simulink model "L13_exercise"  (R2023b)
settings: Solver=FixedStepDiscrete  StartTime=0.0  StopTime=600  FixedStep=0.1  RelTol=1e-3
values from neighbouring files (symbols this model uses):
  Ki = 2    [visualize.m]
  Kp = 1    [visualize.m]
  LP = c2d(tf([N], [1 N]), 0.1)    [visualize.m]
libraries: simulink x8, slpidlib x1
settings Model: PauseTimes=190  Creator=tbcigcb  LastModifiedBy=vojta
settings OptimizationCC: ReuseModelBlockBuffer=off

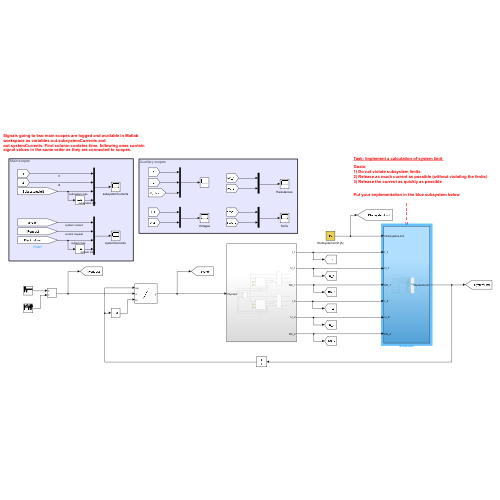
[thumbnail: Simulink's stored preview of the top-level diagram]
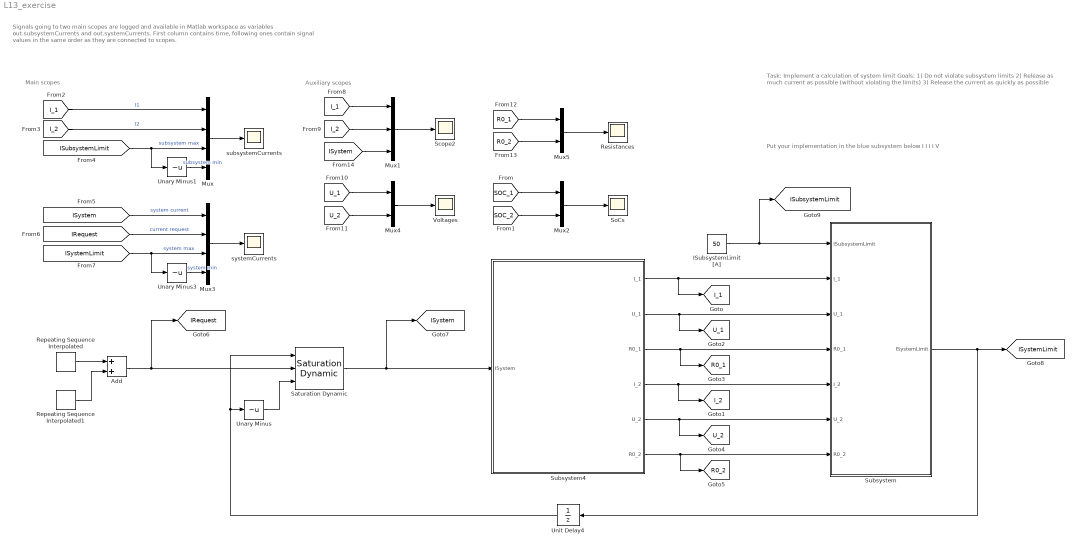
== system L13_exercise ==
  note: Task: Implement a calculation of system limit
      |
      | Goals:
      | 1) Do not violate subsystem limits
      | 2) Release as much current as possible (without violating the limits)
      | 3) Release the current as quickly as possible
  note: Signals going to two main scopes are logged and available in Matlab workspace as variables out.subsystemCurrents and out.systemCurrents. First column contains time, following ones contain signal values in the same order as they are connected to scopes.
  note: Put your implementation in the blue subsystem below
      |
      | I
      | I
      | I
      | I
      | V
  note: Main scopes
  note: Auxiliary scopes
  Add : Sum
  ISubsystemLimit [A] : Constant  Value=50  SampleTime=0.1
  Mux : Mux
  Mux1 : Mux  Inputs=3
  Mux2 : Mux  Inputs=2
  Mux3 : Mux
  Mux4 : Mux  Inputs=2
  Mux5 : Mux  Inputs=2
  Repeating Sequence Interpolated : simulink/Sources/Repeating Sequence Interpolated  OutValues=200*[0 0 1 0 -1 0 0]+0.01  TimeValues=[0 10 20 30 40 50 150]  LookUpMeth=Interpolation-Use End Values  tsamp=0.1  OutMin=[]  OutMax=[]  OutDataTypeStr=double  OutputDataTypeScalingMode=double  OutDataType=fixdt(0,8)  OutScaling=2^-10
  Repeating Sequence Interpolated1 : simulink/Sources/Repeating Sequence Interpolated  OutValues=120*[0 1 0 -1 0 0.5 1 -1 1 0.7 0]+0.01  TimeValues=[0 60 70 80 90 100 110 120 130 140 150]  LookUpMeth=Use Input Below  tsamp=0.1  OutMin=[]  OutMax=[]  OutDataTypeStr=double  OutputDataTypeScalingMode=double  OutDataType=fixdt(0,8)  OutScaling=2^-10
  Resistances : Scope
  Saturation Dynamic : simulink/Discontinuities/Saturation Dynamic  OutMin=[]  OutMax=[]  OutDataTypeStr=Inherit: Same as second input  OutDataType=fixdt(1, 16)  OutScaling=2^-10  DoSatur=off
  Scope2 : Scope
  SoCs : Scope
  Subsystem : Subsystem
  Subsystem4 : Subsystem
  Unary Minus : UnaryMinus
  Unary Minus1 : UnaryMinus
  Unary Minus3 : UnaryMinus
  Unit Delay4 : UnitDelay  InitialCondition=100  SampleTime=-1  HasFrameUpgradeWarning=on
  Voltages : Scope
  subsystemCurrents : Scope
  systemCurrents : Scope
  tag scope: IRequest=global, ISubsystemLimit=global, ISystem=global, ISystemLimit=global, I_1=global, I_2=global, R0_1=global, R0_2=global, U_1=global, U_2=global
  wires:
  Subsystem/1(ISystemLimit) -> [ISystemLimit], Unit Delay4/1
  Unit Delay4/1 -> Saturation Dynamic/1, Unary Minus/1
  Unary Minus/1 -> Saturation Dynamic/3
  Saturation Dynamic/1 -> [ISystem], Subsystem4/1(ISystem)
  Add/1 -> [IRequest], Saturation Dynamic/2
  Mux/1 -> subsystemCurrents/1
  Repeating Sequence Interpolated1/1 -> Add/2
  Repeating Sequence Interpolated/1 -> Add/1
  ISubsystemLimit [A]/1 -> [ISubsystemLimit], Subsystem/1(ISubsystemLimit)
  Unary Minus1/1 -> Mux/4  "subsystem min"
  [SOC_1] -> Mux2/1
  [SOC_2] -> Mux2/2
  Mux2/1 -> SoCs/1
  Subsystem4/1(I_1) -> [I_1], Subsystem/2(I_1)
  Subsystem4/2(U_1) -> [U_1], Subsystem/3(U_1)
  Subsystem4/3(R0_1) -> [R0_1], Subsystem/4(R0_1)
  Subsystem4/4(I_2) -> [I_2], Subsystem/5(I_2)
  Subsystem4/5(U_2) -> [U_2], Subsystem/6(U_2)
  Subsystem4/6(R0_2) -> [R0_2], Subsystem/7(R0_2)
  [I_1] -> Mux/1  "I1"
  [I_2] -> Mux/2  "I2"
  [ISubsystemLimit] -> Unary Minus1/1, Mux/3  "subsystem max"
  Unary Minus3/1 -> Mux3/4  "system min"
  Mux3/1 -> systemCurrents/1
  [IRequest] -> Mux3/2  "current request"
  [ISystemLimit] -> Unary Minus3/1, Mux3/3  "system max"
  [ISystem] -> Mux3/1  "system current"
  Mux1/1 -> Scope2/1
  [I_2] -> Mux1/2
  [I_1] -> Mux1/1
  [U_1] -> Mux4/1
  [U_2] -> Mux4/2
  Mux4/1 -> Voltages/1
  Mux5/1 -> Resistances/1
  [R0_2] -> Mux5/2
  [R0_1] -> Mux5/1
  [ISystem] -> Mux1/3

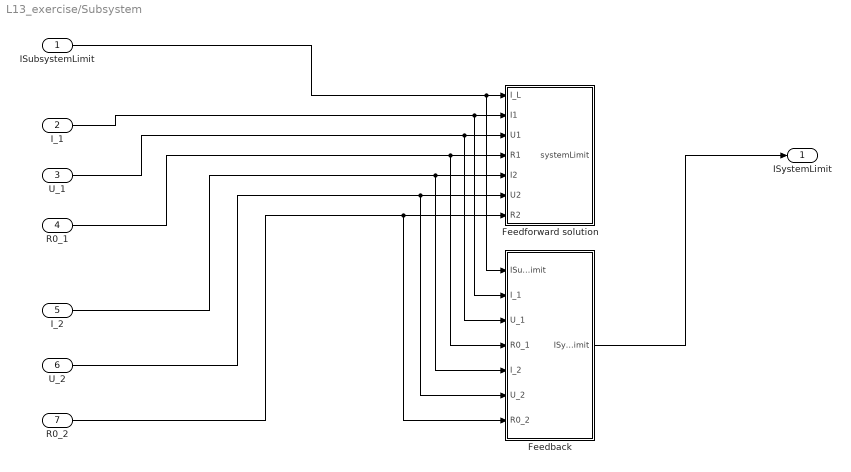
== system L13_exercise/Subsystem ==
  ISubsystemLimit : Inport
  I_1 : Inport  Port=2
  U_1 : Inport  Port=3
  R0_1 : Inport  Port=4
  I_2 : Inport  Port=5
  U_2 : Inport  Port=6
  R0_2 : Inport  Port=7
  Feedback : Subsystem
  Feedforward solution : MATLAB Function  TreatAsAtomicUnit=on
  ISystemLimit : Outport
  wires:
  ISubsystemLimit/1 -> Feedback/1(ISubsystemLimit), Feedforward solution/1(I_L)
  U_1/1 -> Feedback/3(U_1), Feedforward solution/3(U1)
  I_1/1 -> Feedback/2(I_1), Feedforward solution/2(I1)
  R0_1/1 -> Feedback/4(R0_1), Feedforward solution/4(R1)
  I_2/1 -> Feedback/5(I_2), Feedforward solution/5(I2)
  U_2/1 -> Feedback/6(U_2), Feedforward solution/6(U2)
  R0_2/1 -> Feedback/7(R0_2), Feedforward solution/7(R2)
  Feedback/1(ISystemLimit) -> ISystemLimit/1

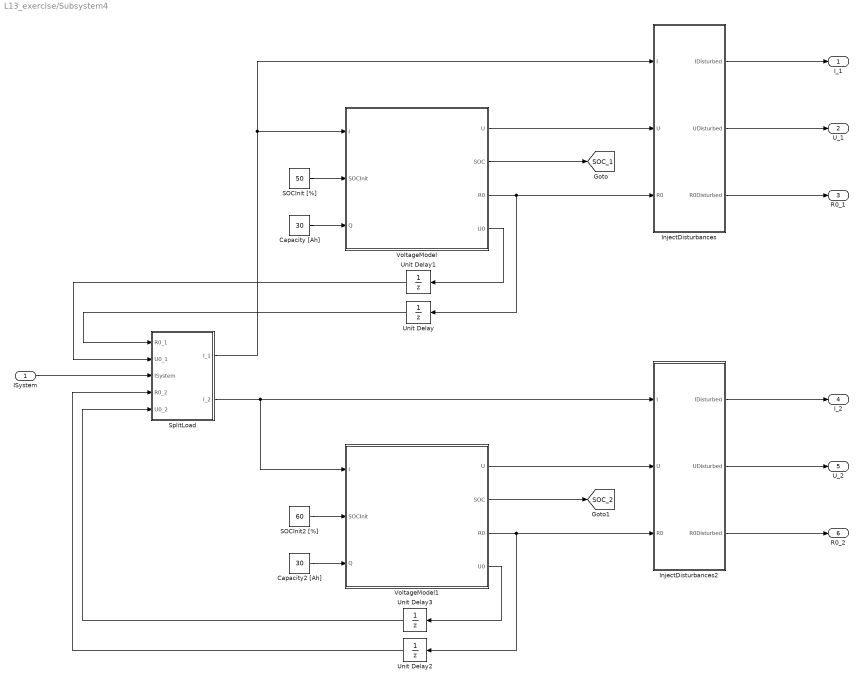
== system L13_exercise/Subsystem4 ==
  ISystem : Inport
  Capacity [Ah] : Constant  Value=30
  Capacity2 [Ah] : Constant  Value=30
  InjectDisturbances : Subsystem
  InjectDisturbances2 : Subsystem
  SOCInit [%] : Constant  Value=50
  SOCInit2 [%] : Constant  Value=60
  SplitLoad : Subsystem
  Unit Delay : UnitDelay  InitialCondition=1  SampleTime=-1  HasFrameUpgradeWarning=on
  Unit Delay1 : UnitDelay  SampleTime=-1  HasFrameUpgradeWarning=on
  Unit Delay2 : UnitDelay  InitialCondition=1  SampleTime=-1  HasFrameUpgradeWarning=on
  Unit Delay3 : UnitDelay  SampleTime=-1  HasFrameUpgradeWarning=on
  VoltageModel : Subsystem
  VoltageModel1 : Subsystem
  I_1 : Outport
  U_1 : Outport  Port=2
  R0_1 : Outport  Port=3
  I_2 : Outport  Port=4
  U_2 : Outport  Port=5
  R0_2 : Outport  Port=6
  tag scope: SOC_1=global, SOC_2=global
  wires:
  SOCInit2 [%]/1 -> VoltageModel1/2(SOCInit)
  SplitLoad/1(I_1) -> InjectDisturbances/1(I), VoltageModel/1(I)
  VoltageModel/4(U0) -> Unit Delay1/1
  Unit Delay1/1 -> SplitLoad/2(U0_1)
  Unit Delay3/1 -> SplitLoad/5(U0_2)
  SplitLoad/2(I_2) -> VoltageModel1/1(I), InjectDisturbances2/1(I)
  Unit Delay/1 -> SplitLoad/1(R0_1)
  VoltageModel1/3(R0) -> InjectDisturbances2/3(R0), Unit Delay2/1
  Unit Delay2/1 -> SplitLoad/4(R0_2)
  SOCInit [%]/1 -> VoltageModel/2(SOCInit)
  VoltageModel/3(R0) -> InjectDisturbances/3(R0), Unit Delay/1
  VoltageModel1/4(U0) -> Unit Delay3/1
  Capacity2 [Ah]/1 -> VoltageModel1/3(Q)
  Capacity [Ah]/1 -> VoltageModel/3(Q)
  ISystem/1 -> SplitLoad/3(ISystem)
  VoltageModel/2(SOC) -> [SOC_1]
  VoltageModel1/2(SOC) -> [SOC_2]
  InjectDisturbances/1(IDisturbed) -> I_1/1
  VoltageModel/1(U) -> InjectDisturbances/2(U)
  InjectDisturbances/2(UDisturbed) -> U_1/1
  InjectDisturbances/3(R0Disturbed) -> R0_1/1
  VoltageModel1/1(U) -> InjectDisturbances2/2(U)
  InjectDisturbances2/3(R0Disturbed) -> R0_2/1
  InjectDisturbances2/2(UDisturbed) -> U_2/1
  InjectDisturbances2/1(IDisturbed) -> I_2/1

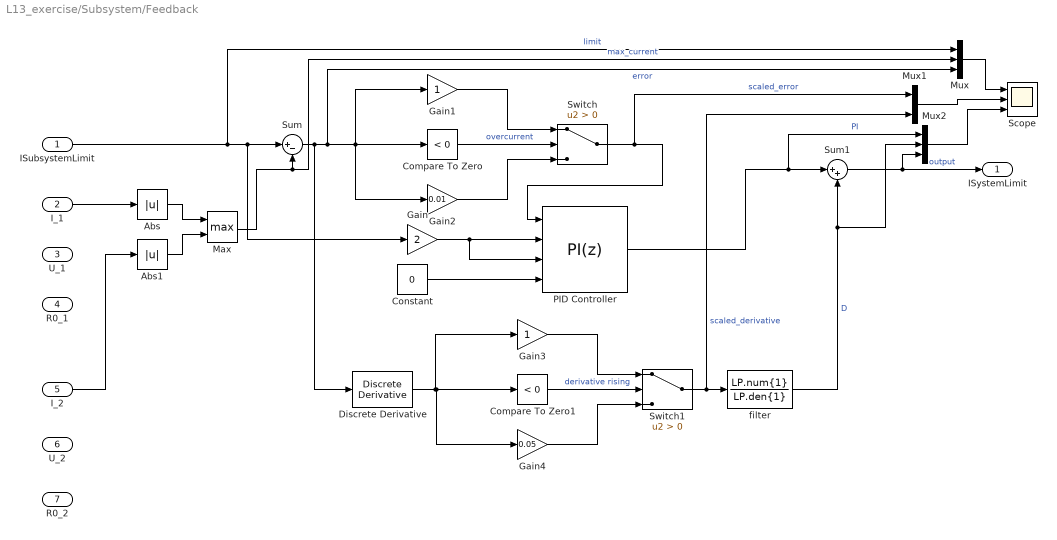
== system L13_exercise/Subsystem/Feedback ==
  ISubsystemLimit : Inport
  I_1 : Inport  Port=2
  U_1 : Inport  Port=3
  R0_1 : Inport  Port=4
  I_2 : Inport  Port=5
  U_2 : Inport  Port=6
  R0_2 : Inport  Port=7
  Abs : Abs  SaturateOnIntegerOverflow=off
  Abs1 : Abs  SaturateOnIntegerOverflow=off
  Compare To Zero : simulink/Logic and Bit Operations/Compare To Zero  relop=<  OutDataTypeStr=boolean
  Compare To Zero1 : simulink/Logic and Bit Operations/Compare To Zero  relop=<  OutDataTypeStr=boolean
  Constant : Constant  Value=0
  Discrete Derivative : simulink/Discrete/Discrete Derivative  gainval=Kd  ICPrevScaledInput=0.0  OutMin=[]  OutMax=[]  OutDataType=fixdt(1, 16)  OutScaling=2^-10  DoSatur=off
  Gain : Gain  Gain=2
  Gain1 : Gain
  Gain2 : Gain  Gain=0.01
  Gain3 : Gain
  Gain4 : Gain  Gain=0.05
  Max : MinMax  Function=max  Inputs=2
  Mux : Mux  Inputs=3
  Mux1 : Mux  Inputs=2
  Mux2 : Mux  Inputs=3
  PID Controller : slpidlib/PID Controller  Controller=PI  Form=Parallel  TimeDomain=Discrete-time  UseExternalTs=off  SampleTime=-1  IntegratorMethod=Forward Euler  FilterMethod=Forward Euler  ControllerParametersSource=internal  P=Kp  I=Ki  UseKiTs=off  D=0  N=100  UseFilter=on  TunerSelectOption=Transfer Function Based (PID Tuner App)  InitialConditionSource=external  InitialConditionForIntegrator=0  InitialConditionForFilter=0  DifferentiatorICPrevScaledInput=0  ExternalReset=none  TrackingMode=off  Kt=1  LimitOutput=on  SatLimitsSource=external  UpperSaturationLimit=inf  LowerSaturationLimit=-inf  LinearizeAsGain=on  AntiWindupMode=clamping  Kb=1  LimitIntegrator=off  UpperIntegratorSaturationLimit=inf  LowerIntegratorSaturationLimit=-inf  POutMin=[]  POutMax=[]  IOutMin=[]  IOutMax=[]  DOutMin=[]  DOutMax=[]  NOutMin=[]  NOutMax=[]  SumOutMin=[]  SumOutMax=[]  SaturationOutMin=[]  SaturationOutMax=[]  PParamMin=[]  PParamMax=[]  IParamMin=[]  IParamMax=[]  DParamMin=[]  DParamMax=[]  NParamMin=[]  NParamMax=[]  KbParamMin=[]  KbParamMax=[]  KtParamMin=[]  KtParamMax=[]  KbOutMin=[]  KbOutMax=[]  KtOutMin=[]  KtOutMax=[]  IntegratorOutMin=[]  IntegratorOutMax=[]  FilterOutMin=[]  FilterOutMax=[]  SumI1OutMin=[]  SumI1OutMax=[]  SumI2OutMin=[]  SumI2OutMax=[]  SumI3OutMin=[]  SumI3OutMax=[]  SumI4OutMin=[]  SumI4OutMax=[]  SumDOutMin=[]  SumDOutMax=[]  DifferentiatorOutMin=[]  DifferentiatorOutMax=[]  FilterDiffOutCoefMin=[]  FilterDiffOutCoefMax=[]  ReciprocalOutMin=[]  ReciprocalOutMax=[]  SumDenOutMin=[]  SumDenOutMax=[]  SumNumOutMin=[]  SumNumOutMax=[]  DivideOutMin=[]  DivideOutMax=[]  UdiffTsProdOutMin=[]  UdiffTsProdOutMax=[]  NTsProdOutMin=[]  NTsProdOutMax=[]  UintegralTsProdOutMin=[]  UintegralTsProdOutMax=[]  UngainTsProdOutMin=[]  UngainTsProdOutMax=[]  ClampingZeroOutDataTypeStr=Inherit: Inherit via back propagation  ClampingZeroOutMin=[]  ClampingZeroOutMax=[]  FilterDenConstantOutDataTypeStr=Inherit: Inherit via back propagation  FilterDenConstantOutMin=[]  FilterDenConstantOutMax=[]  PCopyOutDataTypeStr=Inherit: Inherit via back propagation  PCopyOutMin=[]  PCopyOutMax=[]  NCopyOutDataTypeStr=Inherit: Inherit via back propagation  NCopyOutMin=[]  NCopyOutMax=[]  IntegratorContinuousStateAttributes=''  IntegratorStateMustResolveToSignalObject=off  IntegratorRTWStateStorageClass=Auto  FilterContinuousStateAttributes=''  FilterStateMustResolveToSignalObject=off  FilterRTWStateStorageClass=Auto  ParallelPVariant=InternalParameters  IdealPVariant=Disabled  IVariant=InternalParameters  DVariant=Disabled  IntegratorVariant=Discrete  SatVariant=External  AWVariant=DiscClampingParallel  PCopyVariant=Disabled  TRVariant=Disabled  FdbkBlocksVariant=Forward  IdealPFdbkVariant=Disabled  SatFdbkVariant=Disabled  DerivativeFilterVariant=Disabled  NVariant=Disabled  NCopyVariant=Disabled_SignalSpec  FilterICVariant=Disabled  IntegratorICVariant=ExternalICs  ExternalResetVariant=Disabled  TRSumVariant=Passthrough  SumFdbkVariant=Disabled  SumVariant=Sum_PI  TsampFilterVariant=InternalTs  TsampNgainVariant=Passthrough  TsampIntegralVariant=Disabled_SignalSpec  ExternalSaturationOutDataTypeStr=Inherit: Same as second input
  Scope : Scope  NumInputPorts=3
  Sum : Sum  Inputs=|+-
  Sum1 : Sum  Inputs=|++
  Switch : Switch  Criteria=u2 > Threshold  SaturateOnIntegerOverflow=off  InputSameDT=off
  Switch1 : Switch  Criteria=u2 > Threshold  SaturateOnIntegerOverflow=off  InputSameDT=off
  filter : DiscreteTransferFcn  Numerator=LP.num{1}  Denominator=LP.den{1}
  ISystemLimit : Outport
  wires:
  I_1/1 -> Abs/1
  I_2/1 -> Abs1/1
  Abs/1 -> Max/1
  Abs1/1 -> Max/2
  ISubsystemLimit/1 -> Mux/1, Gain/1, Sum/1  "limit"
  Max/1 -> Sum/2, Mux/2  "max_current"
  Sum1/1 -> Mux2/3, ISystemLimit/1  "output"
  Constant/1 -> PID Controller/4
  Gain/1 -> PID Controller/2, PID Controller/3
  Sum/1 -> Discrete Derivative/1, Mux/3, Gain2/1, Gain1/1, Compare To Zero/1  "error"
  Compare To Zero/1 -> Switch/2  "overcurrent"
  Switch/1 -> Mux1/1, PID Controller/1  "scaled_error"
  Gain2/1 -> Switch/3
  Gain1/1 -> Switch/1
  PID Controller/1 -> Mux2/1, Sum1/1  "PI"
  filter/1 -> Mux2/2, Sum1/2  "D"
  Compare To Zero1/1 -> Switch1/2  "derivative rising"
  Discrete Derivative/1 -> Gain3/1, Gain4/1, Compare To Zero1/1
  Gain4/1 -> Switch1/3
  Gain3/1 -> Switch1/1
  Switch1/1 -> Mux1/2, filter/1  "scaled_derivative"
  Mux/1 -> Scope/1
  Mux1/1 -> Scope/2
  Mux2/1 -> Scope/3

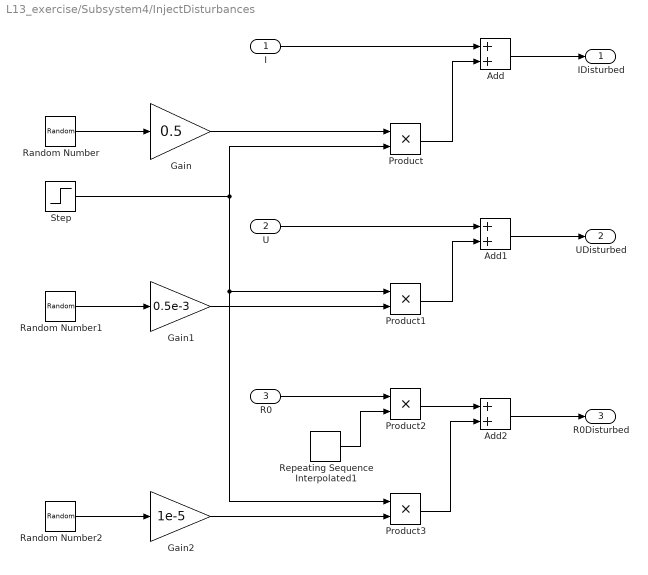
== system L13_exercise/Subsystem4/InjectDisturbances ==
  I : Inport
  U : Inport  Port=2
  R0 : Inport  Port=3
  Add : Sum
  Add1 : Sum
  Add2 : Sum
  Gain : Gain  Gain=0.5
  Gain1 : Gain  Gain=0.5e-3
  Gain2 : Gain  Gain=1e-5
  Product{,1..3} (4 alike) : Product
  Random Number : RandomNumber  SampleTime=0.1
  Random Number1 : RandomNumber  Seed=1  SampleTime=0.1
  Random Number2 : RandomNumber  Seed=2  SampleTime=0.1
  Repeating Sequence Interpolated1 : simulink/Sources/Repeating Sequence Interpolated  OutValues=[1 1 0.9 1.1 1]  TimeValues=[0 150 300 450 600]  LookUpMeth=Use Input Below  tsamp=0.1  OutMin=[]  OutMax=[]  OutDataTypeStr=double  OutputDataTypeScalingMode=double  OutDataType=fixdt(0,8)  OutScaling=2^-10
  Step : Step  Time=150  SampleTime=0.1
  IDisturbed : Outport
  UDisturbed : Outport  Port=2
  R0Disturbed : Outport  Port=3
  wires:
  Random Number1/1 -> Gain1/1
  Random Number/1 -> Gain/1
  I/1 -> Add/1
  Add/1 -> IDisturbed/1
  U/1 -> Add1/1
  Add1/1 -> UDisturbed/1
  Step/1 -> Product3/1, Product1/1, Product/2
  Gain/1 -> Product/1
  Product/1 -> Add/2
  Gain1/1 -> Product1/2
  Product1/1 -> Add1/2
  R0/1 -> Product2/1
  Repeating Sequence Interpolated1/1 -> Product2/2
  Random Number2/1 -> Gain2/1
  Product2/1 -> Add2/1
  Add2/1 -> R0Disturbed/1
  Gain2/1 -> Product3/2
  Product3/1 -> Add2/2

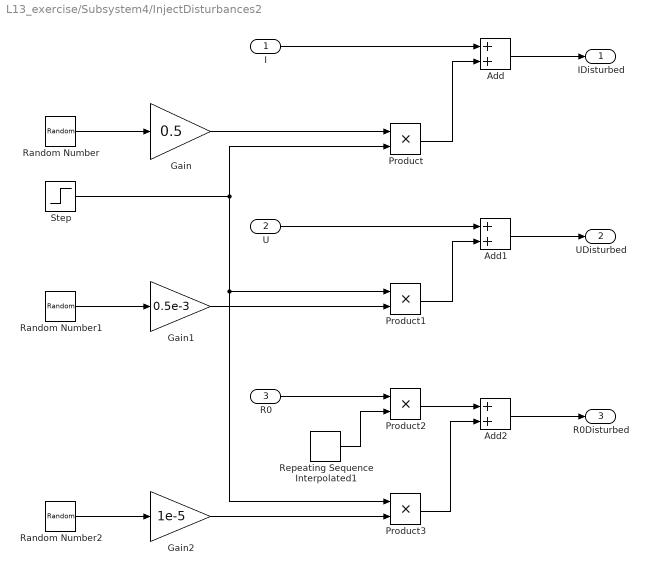
== system L13_exercise/Subsystem4/InjectDisturbances2 ==
  I : Inport
  U : Inport  Port=2
  R0 : Inport  Port=3
  Add : Sum
  Add1 : Sum
  Add2 : Sum
  Gain : Gain  Gain=0.5
  Gain1 : Gain  Gain=0.5e-3
  Gain2 : Gain  Gain=1e-5
  Product{,1..3} (4 alike) : Product
  Random Number : RandomNumber  Seed=3  SampleTime=0.1
  Random Number1 : RandomNumber  Seed=5  SampleTime=0.1
  Random Number2 : RandomNumber  Seed=7  SampleTime=0.1
  Repeating Sequence Interpolated1 : simulink/Sources/Repeating Sequence Interpolated  OutValues=[1 1 0.7 1.4 1]  TimeValues=[0 150 300 450 600]  LookUpMeth=Use Input Below  tsamp=0.1  OutMin=[]  OutMax=[]  OutDataTypeStr=double  OutputDataTypeScalingMode=double  OutDataType=fixdt(0,8)  OutScaling=2^-10
  Step : Step  Time=150  SampleTime=0.1
  IDisturbed : Outport
  UDisturbed : Outport  Port=2
  R0Disturbed : Outport  Port=3
  wires:
  Product3/1 -> Add2/2
  Gain2/1 -> Product3/2
  Add2/1 -> R0Disturbed/1
  Product2/1 -> Add2/1
  Random Number2/1 -> Gain2/1
  Repeating Sequence Interpolated1/1 -> Product2/2
  R0/1 -> Product2/1
  Product1/1 -> Add1/2
  Gain1/1 -> Product1/2
  Product/1 -> Add/2
  Gain/1 -> Product/1
  Step/1 -> Product/2, Product1/1, Product3/1
  Add1/1 -> UDisturbed/1
  U/1 -> Add1/1
  Add/1 -> IDisturbed/1
  I/1 -> Add/1
  Random Number/1 -> Gain/1
  Random Number1/1 -> Gain1/1

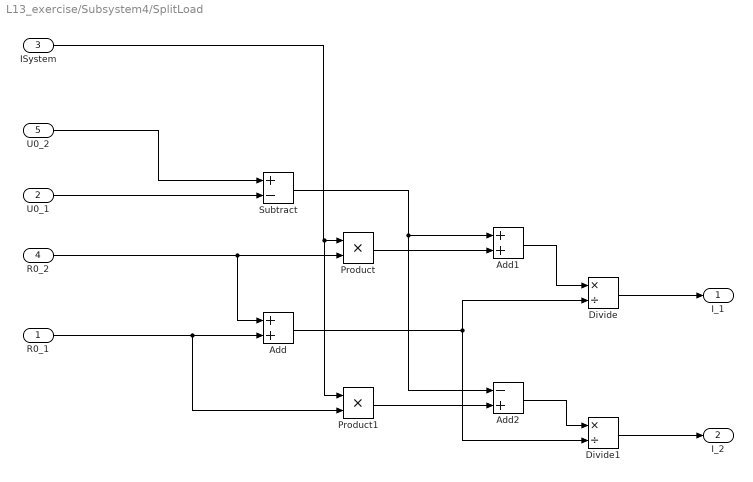
== system L13_exercise/Subsystem4/SplitLoad ==
  R0_1 : Inport
  U0_1 : Inport  Port=2
  ISystem : Inport  Port=3
  R0_2 : Inport  Port=4
  U0_2 : Inport  Port=5
  Add : Sum
  Add1 : Sum
  Add2 : Sum  Inputs=-+
  Divide : Product  Inputs=*/
  Divide1 : Product  Inputs=*/
  Product : Product
  Product1 : Product
  Subtract : Sum  Inputs=+-
  I_1 : Outport
  I_2 : Outport  Port=2
  wires:
  R0_2/1 -> Add/1, Product/2
  R0_1/1 -> Product1/2, Add/2
  U0_2/1 -> Subtract/1
  U0_1/1 -> Subtract/2
  ISystem/1 -> Product1/1, Product/1
  Subtract/1 -> Add2/1, Add1/1
  Product/1 -> Add1/2
  Add1/1 -> Divide/1
  Add/1 -> Divide/2, Divide1/2
  Divide/1 -> I_1/1
  Product1/1 -> Add2/2
  Add2/1 -> Divide1/1
  Divide1/1 -> I_2/1

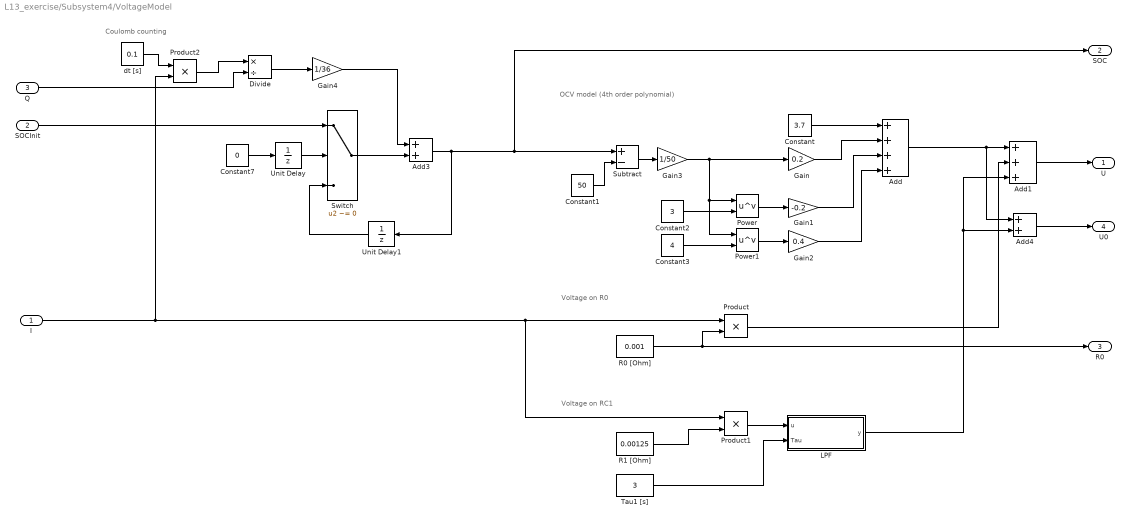
== system L13_exercise/Subsystem4/VoltageModel ==
  note: Voltage on RC1
  note: Voltage on R0
  note: OCV model (4th order polynomial)
  note: Coulomb counting
  I : Inport
  SOCInit : Inport  Port=2
  Q : Inport  Port=3
  Add : Sum  Inputs=++++
  Add1 : Sum  Inputs=+++
  Add3 : Sum
  Add4 : Sum
  Constant : Constant  Value=3.7
  Constant1 : Constant  Value=50
  Constant2 : Constant  Value=3
  Constant3 : Constant  Value=4
  Constant7 : Constant  Value=0
  Divide : Product  Inputs=*/
  Gain : Gain  Gain=0.2
  Gain1 : Gain  Gain=-0.2
  Gain2 : Gain  Gain=0.4
  Gain3 : Gain  Gain=1/50
  Gain4 : Gain  Gain=1/36
  LPF : Subsystem
  Power : Math  Operator=pow
  Power1 : Math  Operator=pow
  Product : Product
  Product1 : Product
  Product2 : Product
  R0 [Ohm] : Constant  Value=0.001
  R1 [Ohm] : Constant  Value=0.00125
  Subtract : Sum  Inputs=+-
  Switch : Switch  Criteria=u2 ~= 0  SaturateOnIntegerOverflow=off  InputSameDT=off
  Tau1 [s] : Constant  Value=3
  Unit Delay : UnitDelay  InitialCondition=1  SampleTime=-1  HasFrameUpgradeWarning=on
  Unit Delay1 : UnitDelay  InitialCondition=1  SampleTime=-1  HasFrameUpgradeWarning=on
  dt [s] : Constant  Value=0.1
  U : Outport
  SOC : Outport  Port=2
  R0 : Outport  Port=3
  U0 : Outport  Port=4
  wires:
  Constant1/1 -> Subtract/2
  Subtract/1 -> Gain3/1
  Gain3/1 -> Power1/1, Power/1, Gain/1
  Power/1 -> Gain1/1
  Constant/1 -> Add/1
  Gain/1 -> Add/2
  Gain1/1 -> Add/3
  Gain2/1 -> Add/4
  Constant2/1 -> Power/2
  Constant3/1 -> Power1/2
  Power1/1 -> Gain2/1
  I/1 -> Product/1, Product1/1, Product2/2
  R0 [Ohm]/1 -> Product/2, R0/1
  R1 [Ohm]/1 -> Product1/2
  Product1/1 -> LPF/1(u)
  Add/1 -> Add4/1, Add1/1
  LPF/1(y) -> Add4/2, Add1/3
  Add1/1 -> U/1
  Tau1 [s]/1 -> LPF/2(Tau)
  Add4/1 -> U0/1
  Constant7/1 -> Unit Delay/1
  Unit Delay/1 -> Switch/2
  SOCInit/1 -> Switch/1
  dt [s]/1 -> Product2/1
  Unit Delay1/1 -> Switch/3
  Product2/1 -> Divide/1
  Q/1 -> Divide/2
  Divide/1 -> Gain4/1
  Switch/1 -> Add3/2
  Add3/1 -> SOC/1, Subtract/1, Unit Delay1/1
  Gain4/1 -> Add3/1
  Product/1 -> Add1/2

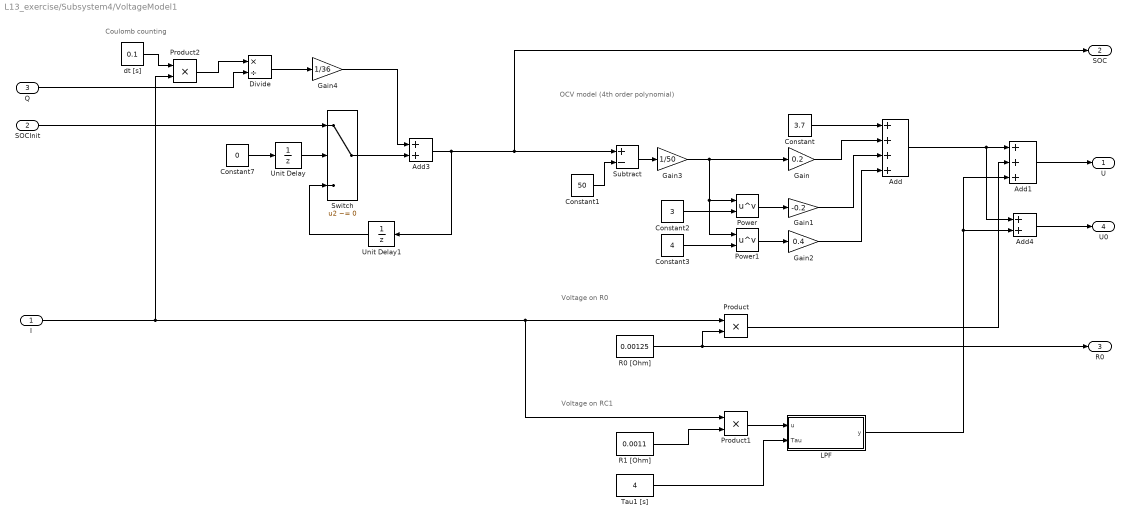
== system L13_exercise/Subsystem4/VoltageModel1 ==
  note: Coulomb counting
  note: OCV model (4th order polynomial)
  note: Voltage on R0
  note: Voltage on RC1
  I : Inport
  SOCInit : Inport  Port=2
  Q : Inport  Port=3
  Add : Sum  Inputs=++++
  Add1 : Sum  Inputs=+++
  Add3 : Sum
  Add4 : Sum
  Constant : Constant  Value=3.7
  Constant1 : Constant  Value=50
  Constant2 : Constant  Value=3
  Constant3 : Constant  Value=4
  Constant7 : Constant  Value=0
  Divide : Product  Inputs=*/
  Gain : Gain  Gain=0.2
  Gain1 : Gain  Gain=-0.2
  Gain2 : Gain  Gain=0.4
  Gain3 : Gain  Gain=1/50
  Gain4 : Gain  Gain=1/36
  LPF : Subsystem
  Power : Math  Operator=pow
  Power1 : Math  Operator=pow
  Product : Product
  Product1 : Product
  Product2 : Product
  R0 [Ohm] : Constant  Value=0.00125
  R1 [Ohm] : Constant  Value=0.0011
  Subtract : Sum  Inputs=+-
  Switch : Switch  Criteria=u2 ~= 0  SaturateOnIntegerOverflow=off  InputSameDT=off
  Tau1 [s] : Constant  Value=4
  Unit Delay : UnitDelay  InitialCondition=1  SampleTime=-1  HasFrameUpgradeWarning=on
  Unit Delay1 : UnitDelay  InitialCondition=1  SampleTime=-1  HasFrameUpgradeWarning=on
  dt [s] : Constant  Value=0.1
  U : Outport
  SOC : Outport  Port=2
  R0 : Outport  Port=3
  U0 : Outport  Port=4
  wires:
  Product/1 -> Add1/2
  Gain4/1 -> Add3/1
  Add3/1 -> Unit Delay1/1, Subtract/1, SOC/1
  Switch/1 -> Add3/2
  Divide/1 -> Gain4/1
  Q/1 -> Divide/2
  Product2/1 -> Divide/1
  Unit Delay1/1 -> Switch/3
  dt [s]/1 -> Product2/1
  SOCInit/1 -> Switch/1
  Unit Delay/1 -> Switch/2
  Constant7/1 -> Unit Delay/1
  Add4/1 -> U0/1
  Tau1 [s]/1 -> LPF/2(Tau)
  Add1/1 -> U/1
  LPF/1(y) -> Add1/3, Add4/2
  Add/1 -> Add1/1, Add4/1
  Product1/1 -> LPF/1(u)
  R1 [Ohm]/1 -> Product1/2
  R0 [Ohm]/1 -> R0/1, Product/2
  I/1 -> Product2/2, Product1/1, Product/1
  Power1/1 -> Gain2/1
  Constant3/1 -> Power1/2
  Constant2/1 -> Power/2
  Gain2/1 -> Add/4
  Gain1/1 -> Add/3
  Gain/1 -> Add/2
  Constant/1 -> Add/1
  Power/1 -> Gain1/1
  Gain3/1 -> Gain/1, Power/1, Power1/1
  Subtract/1 -> Gain3/1
  Constant1/1 -> Subtract/2

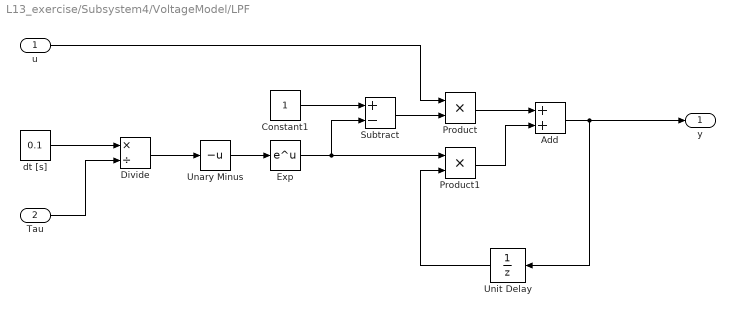
== system L13_exercise/Subsystem4/VoltageModel/LPF ==
  u : Inport
  Tau : Inport  Port=2
  Add : Sum
  Constant1 : Constant
  Divide : Product  Inputs=*/
  Exp : Math
  Product : Product
  Product1 : Product
  Subtract : Sum  Inputs=+-
  Unary Minus : UnaryMinus
  Unit Delay : UnitDelay  SampleTime=-1  HasFrameUpgradeWarning=on
  dt [s] : Constant  Value=0.1
  y : Outport
  wires:
  dt [s]/1 -> Divide/1
  Tau/1 -> Divide/2
  Divide/1 -> Unary Minus/1
  Unary Minus/1 -> Exp/1
  Exp/1 -> Subtract/2, Product1/1
  Unit Delay/1 -> Product1/2
  Constant1/1 -> Subtract/1
  u/1 -> Product/1
  Subtract/1 -> Product/2
  Product/1 -> Add/1
  Product1/1 -> Add/2
  Add/1 -> Unit Delay/1, y/1

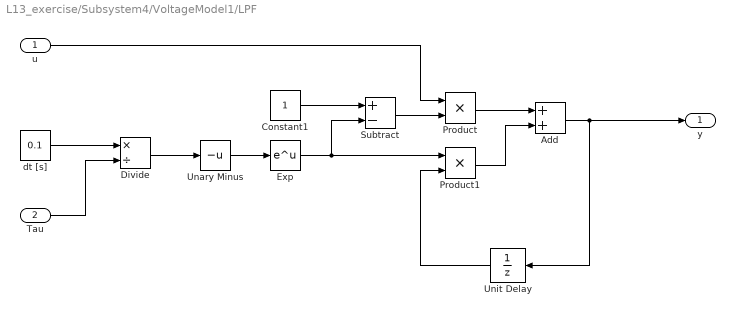
== system L13_exercise/Subsystem4/VoltageModel1/LPF ==
  u : Inport
  Tau : Inport  Port=2
  Add : Sum
  Constant1 : Constant
  Divide : Product  Inputs=*/
  Exp : Math
  Product : Product
  Product1 : Product
  Subtract : Sum  Inputs=+-
  Unary Minus : UnaryMinus
  Unit Delay : UnitDelay  SampleTime=-1  HasFrameUpgradeWarning=on
  dt [s] : Constant  Value=0.1
  y : Outport
  wires:
  Add/1 -> y/1, Unit Delay/1
  Product1/1 -> Add/2
  Product/1 -> Add/1
  Subtract/1 -> Product/2
  u/1 -> Product/1
  Constant1/1 -> Subtract/1
  Unit Delay/1 -> Product1/2
  Exp/1 -> Product1/1, Subtract/2
  Unary Minus/1 -> Exp/1
  Divide/1 -> Unary Minus/1
  Tau/1 -> Divide/2
  dt [s]/1 -> Divide/1

== matlab function L13_exercise/Subsystem/Feedforward solution ==
  data: I_L input; systemLimit output; I1 input; U1 input; R1 input; I2 input; U2 input; R2 input
function systemLimit = fun(I_L, I1, U1, R1, I2, U2, R2)
[systemLimit, ~] = getSystemCurrentLimit(I_L, [I1, I2], [U1 U2], [R1 R2]);
